simulink subsystem "Gravity_and_Propulsion"  (R2024b)
settings: Solver=VariableStepAuto  StartTime=0.0  StopTime=10.0  RelTol=1e-3
values from neighbouring files (symbols this model uses):
  F_thrust = [114.957 344.87 574.783 2216.543 5270.148 7017.697 7459.19 7900.683 8061.78 7942.48 7842.183 7760.89 ... (1300 elements, 1300x1)]    [barrowaman.mat]
  mass = [57.02 56.99 56.96 56.91 56.87 56.84 56.81 56.78 56.73 56.69 56.66 56.63 ... (1300 elements, 1300x1)]    [barrowaman.mat]
  sim_time = [0.01 0.02 0.03 0.04 0.05 0.06 0.07 0.08 0.09 0.1 0.11 0.12 ... (1300 elements, 1300x1)]    [barrowaman.mat]
settings Model: Creator=joedo  LastModifiedBy=joedo

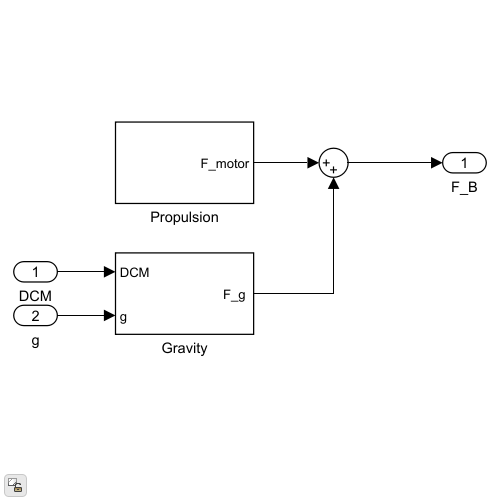
[thumbnail: Simulink's stored preview of the top-level diagram]
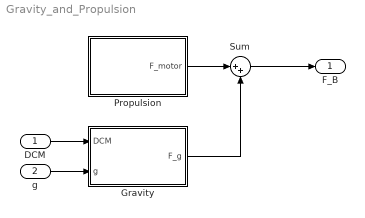
== system Gravity_and_Propulsion ==
  DCM : Inport
  g : Inport  Port=2
  "Gravity " : Subsystem
  "Propulsion " : Subsystem
  Sum : Sum  Inputs=|++
  F_B : Outport  VectorParamsAs1DForOutWhenUnconnected=off
  wires:
  Sum/1 -> F_B/1
  "Propulsion "/1(F_motor) -> Sum/1
  DCM/1 -> "Gravity "/1(DCM)
  "Gravity "/1("F_g ") -> Sum/2
  g/1 -> "Gravity "/2(g)

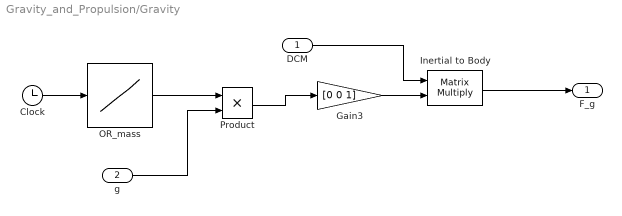
== system Gravity_and_Propulsion/Gravity  ==
  DCM : Inport
  g : Inport  Port=2
  Clock : Clock
  Gain3 : Gain  Gain=[0 0 1]
  Inertial to Body : Product  Multiplication=Matrix(*)  InputSameDT=on  SaturateOnIntegerOverflow=on  OutDataTypeStr=Inherit: Same as first input
  OR_mass : Lookup_n-D  NumberOfTableDimensions=1  BreakpointsForDimension1=sim_time  Table=mass  InternalRulePriority=Speed  RndMeth=Simplest
  Product : Product
  "F_g " : Outport  VectorParamsAs1DForOutWhenUnconnected=off
  wires:
  g/1 -> Product/2
  Clock/1 -> OR_mass/1
  Product/1 -> Gain3/1
  OR_mass/1 -> Product/1
  Gain3/1 -> Inertial to Body/2
  DCM/1 -> Inertial to Body/1
  Inertial to Body/1 -> "F_g "/1

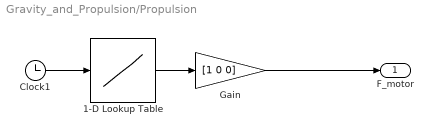
== system Gravity_and_Propulsion/Propulsion  ==
  1-D Lookup Table : Lookup_n-D  NumberOfTableDimensions=1  BreakpointsForDimension1=sim_time  Table=F_thrust  InternalRulePriority=Speed  RndMeth=Simplest
  Clock1 : Clock
  Gain : Gain  Gain=[1 0 0]
  F_motor : Outport  VectorParamsAs1DForOutWhenUnconnected=off
  wires:
  Gain/1 -> F_motor/1
  1-D Lookup Table/1 -> Gain/1
  Clock1/1 -> 1-D Lookup Table/1
